simulink model "BatteryFarmTemplate"  (R2022b)
settings: Solver=VariableStepAuto  StartTime=0.0  StopTime=10.0  RelTol=1e-3  AbsTol=1e-3  EnableMultiTasking=on
libraries: ee_lib x242, sdl_lib x84, fl_lib x43
(part 2 of 5)

== system BatteryFarmTemplate/Battery Conex 1/Battery Charger 3 ==
  DC Voltage Source : fl_lib/Electrical/Electrical Sources/DC Voltage Source  v0=24 V
  DC Voltage Source1 : fl_lib/Electrical/Electrical Sources/DC Voltage Source  v0=24 V
  DC Voltage Source2 : fl_lib/Electrical/Electrical Sources/DC Voltage Source  v0=24 V
  SPST Relay : ee_lib/Switches & Breakers/Relays/SPST Relay  block_choices=ee.enum.controlport.ps  R_closed=0.01 Ohm  G_open=1e-8 1/Ohm  Threshold=0  exposemeasurement=ee.enum.exposemeasurement.hidden  V_rated=5 V  V_energize=75  V_deenergize=25  l_winding=0.08 H  r_winding=12.5 Ohm  g_winding=1e-9 1/Ohm  T_brk_C_S=0 s  T_mak_C_S=0 s  enable_faults=ee.enum.relays.enable.no  fault_action=ee.enum.relays.faultaction.none  fault_types=ee.enum.relays.faultTypes.winding  fault_condition_ps=ee.enum.relays.faultConditionSPSTps.csstuck  r_deg_closed_s=1e-9 Ohm  winding_tau_fault=1e-3 s  tau_fault=1e-3 s  enable_temporal_fault=ee.enum.relays.enable.no  t_fault_stick=1 s  t_fault_ComOpen=1 s  t_fault=1 s  enable_behavioral_fault=ee.enum.relays.enable.no  winding_max_permissible_voltage=inf V  n_fail_on_voltage=1  winding_max_permissible_current=inf A  max_permissible_current=inf A  t_fail_on_current=1 s
      settings: InternalSimscapePortConfiguration="{\"Bottom\":[],\"Left\":[{\"id\":\"PS\",\"label\":\"PS\",\"type\":\"input\"}],\"Right\":[{\"id\":\"S\",\"label\":\"S\",\"type\":\"foundation.electrical.electrical\"},{\"id\":\"COM\",\"label\":\"C\",\"type\":\"foundation.electrical.electrical\"}],\"Top\":[]}"
  SPST Relay1 : ee_lib/Switches & Breakers/Relays/SPST Relay  block_choices=ee.enum.controlport.ps  R_closed=0.01 Ohm  G_open=1e-8 1/Ohm  Threshold=0  exposemeasurement=ee.enum.exposemeasurement.hidden  V_rated=5 V  V_energize=75  V_deenergize=25  l_winding=0.08 H  r_winding=12.5 Ohm  g_winding=1e-9 1/Ohm  T_brk_C_S=0 s  T_mak_C_S=0 s  enable_faults=ee.enum.relays.enable.no  fault_action=ee.enum.relays.faultaction.none  fault_types=ee.enum.relays.faultTypes.winding  fault_condition_ps=ee.enum.relays.faultConditionSPSTps.csstuck  r_deg_closed_s=1e-9 Ohm  winding_tau_fault=1e-3 s  tau_fault=1e-3 s  enable_temporal_fault=ee.enum.relays.enable.no  t_fault_stick=1 s  t_fault_ComOpen=1 s  t_fault=1 s  enable_behavioral_fault=ee.enum.relays.enable.no  winding_max_permissible_voltage=inf V  n_fail_on_voltage=1  winding_max_permissible_current=inf A  max_permissible_current=inf A  t_fail_on_current=1 s
      settings: InternalSimscapePortConfiguration="{\"Bottom\":[],\"Left\":[{\"id\":\"PS\",\"label\":\"PS\",\"type\":\"input\"}],\"Right\":[{\"id\":\"S\",\"label\":\"S\",\"type\":\"foundation.electrical.electrical\"},{\"id\":\"COM\",\"label\":\"C\",\"type\":\"foundation.electrical.electrical\"}],\"Top\":[]}"
  SPST Relay2 : ee_lib/Switches & Breakers/Relays/SPST Relay  block_choices=ee.enum.controlport.ps  R_closed=0.01 Ohm  G_open=1e-8 1/Ohm  Threshold=0  exposemeasurement=ee.enum.exposemeasurement.hidden  V_rated=5 V  V_energize=75  V_deenergize=25  l_winding=0.08 H  r_winding=12.5 Ohm  g_winding=1e-9 1/Ohm  T_brk_C_S=0 s  T_mak_C_S=0 s  enable_faults=ee.enum.relays.enable.no  fault_action=ee.enum.relays.faultaction.none  fault_types=ee.enum.relays.faultTypes.winding  fault_condition_ps=ee.enum.relays.faultConditionSPSTps.csstuck  r_deg_closed_s=1e-9 Ohm  winding_tau_fault=1e-3 s  tau_fault=1e-3 s  enable_temporal_fault=ee.enum.relays.enable.no  t_fault_stick=1 s  t_fault_ComOpen=1 s  t_fault=1 s  enable_behavioral_fault=ee.enum.relays.enable.no  winding_max_permissible_voltage=inf V  n_fail_on_voltage=1  winding_max_permissible_current=inf A  max_permissible_current=inf A  t_fail_on_current=1 s
      settings: InternalSimscapePortConfiguration="{\"Bottom\":[],\"Left\":[{\"id\":\"PS\",\"label\":\"PS\",\"type\":\"input\"}],\"Right\":[{\"id\":\"S\",\"label\":\"S\",\"type\":\"foundation.electrical.electrical\"},{\"id\":\"COM\",\"label\":\"C\",\"type\":\"foundation.electrical.electrical\"}],\"Top\":[]}"
  In 1 : PMIOPort  Side=Left
  Out 1 : PMIOPort  Port=2  Side=Left
  In 2 : PMIOPort  Port=3  Side=Left
  Out 2 : PMIOPort  Port=4  Side=Left
  In 3 : PMIOPort  Port=5  Side=Left
  Out 3 : PMIOPort  Port=6  Side=Left
  Energerize Battery Charger : PMIOPort  Port=7  Side=Right
  connections:
  DC Voltage Source/LConn1 -- SPST Relay/RConn1
  SPST Relay/RConn2 -- In 1/RConn1
  DC Voltage Source/RConn1 -- Out 1/RConn1
  DC Voltage Source1/RConn1 -- Out 2/RConn1
  DC Voltage Source1/LConn1 -- SPST Relay1/RConn1
  SPST Relay1/RConn2 -- In 2/RConn1
  DC Voltage Source2/RConn1 -- Out 3/RConn1
  DC Voltage Source2/LConn1 -- SPST Relay2/RConn1
  SPST Relay2/RConn2 -- In 3/RConn1
  SPST Relay1/LConn1 -- Energerize Battery Charger/RConn1 -- SPST Relay/LConn1 -- SPST Relay2/LConn1

== system BatteryFarmTemplate/Battery Conex 1/Battery Charger 4 ==
  DC Voltage Source : fl_lib/Electrical/Electrical Sources/DC Voltage Source  v0=24 V
  DC Voltage Source1 : fl_lib/Electrical/Electrical Sources/DC Voltage Source  v0=24 V
  DC Voltage Source2 : fl_lib/Electrical/Electrical Sources/DC Voltage Source  v0=24 V
  SPST Relay : ee_lib/Switches & Breakers/Relays/SPST Relay  block_choices=ee.enum.controlport.ps  R_closed=0.01 Ohm  G_open=1e-8 1/Ohm  Threshold=0  exposemeasurement=ee.enum.exposemeasurement.hidden  V_rated=5 V  V_energize=75  V_deenergize=25  l_winding=0.08 H  r_winding=12.5 Ohm  g_winding=1e-9 1/Ohm  T_brk_C_S=0 s  T_mak_C_S=0 s  enable_faults=ee.enum.relays.enable.no  fault_action=ee.enum.relays.faultaction.none  fault_types=ee.enum.relays.faultTypes.winding  fault_condition_ps=ee.enum.relays.faultConditionSPSTps.csstuck  r_deg_closed_s=1e-9 Ohm  winding_tau_fault=1e-3 s  tau_fault=1e-3 s  enable_temporal_fault=ee.enum.relays.enable.no  t_fault_stick=1 s  t_fault_ComOpen=1 s  t_fault=1 s  enable_behavioral_fault=ee.enum.relays.enable.no  winding_max_permissible_voltage=inf V  n_fail_on_voltage=1  winding_max_permissible_current=inf A  max_permissible_current=inf A  t_fail_on_current=1 s
      settings: InternalSimscapePortConfiguration="{\"Bottom\":[],\"Left\":[{\"id\":\"PS\",\"label\":\"PS\",\"type\":\"input\"}],\"Right\":[{\"id\":\"S\",\"label\":\"S\",\"type\":\"foundation.electrical.electrical\"},{\"id\":\"COM\",\"label\":\"C\",\"type\":\"foundation.electrical.electrical\"}],\"Top\":[]}"
  SPST Relay1 : ee_lib/Switches & Breakers/Relays/SPST Relay  block_choices=ee.enum.controlport.ps  R_closed=0.01 Ohm  G_open=1e-8 1/Ohm  Threshold=0  exposemeasurement=ee.enum.exposemeasurement.hidden  V_rated=5 V  V_energize=75  V_deenergize=25  l_winding=0.08 H  r_winding=12.5 Ohm  g_winding=1e-9 1/Ohm  T_brk_C_S=0 s  T_mak_C_S=0 s  enable_faults=ee.enum.relays.enable.no  fault_action=ee.enum.relays.faultaction.none  fault_types=ee.enum.relays.faultTypes.winding  fault_condition_ps=ee.enum.relays.faultConditionSPSTps.csstuck  r_deg_closed_s=1e-9 Ohm  winding_tau_fault=1e-3 s  tau_fault=1e-3 s  enable_temporal_fault=ee.enum.relays.enable.no  t_fault_stick=1 s  t_fault_ComOpen=1 s  t_fault=1 s  enable_behavioral_fault=ee.enum.relays.enable.no  winding_max_permissible_voltage=inf V  n_fail_on_voltage=1  winding_max_permissible_current=inf A  max_permissible_current=inf A  t_fail_on_current=1 s
      settings: InternalSimscapePortConfiguration="{\"Bottom\":[],\"Left\":[{\"id\":\"PS\",\"label\":\"PS\",\"type\":\"input\"}],\"Right\":[{\"id\":\"S\",\"label\":\"S\",\"type\":\"foundation.electrical.electrical\"},{\"id\":\"COM\",\"label\":\"C\",\"type\":\"foundation.electrical.electrical\"}],\"Top\":[]}"
  SPST Relay2 : ee_lib/Switches & Breakers/Relays/SPST Relay  block_choices=ee.enum.controlport.ps  R_closed=0.01 Ohm  G_open=1e-8 1/Ohm  Threshold=0  exposemeasurement=ee.enum.exposemeasurement.hidden  V_rated=5 V  V_energize=75  V_deenergize=25  l_winding=0.08 H  r_winding=12.5 Ohm  g_winding=1e-9 1/Ohm  T_brk_C_S=0 s  T_mak_C_S=0 s  enable_faults=ee.enum.relays.enable.no  fault_action=ee.enum.relays.faultaction.none  fault_types=ee.enum.relays.faultTypes.winding  fault_condition_ps=ee.enum.relays.faultConditionSPSTps.csstuck  r_deg_closed_s=1e-9 Ohm  winding_tau_fault=1e-3 s  tau_fault=1e-3 s  enable_temporal_fault=ee.enum.relays.enable.no  t_fault_stick=1 s  t_fault_ComOpen=1 s  t_fault=1 s  enable_behavioral_fault=ee.enum.relays.enable.no  winding_max_permissible_voltage=inf V  n_fail_on_voltage=1  winding_max_permissible_current=inf A  max_permissible_current=inf A  t_fail_on_current=1 s
      settings: InternalSimscapePortConfiguration="{\"Bottom\":[],\"Left\":[{\"id\":\"PS\",\"label\":\"PS\",\"type\":\"input\"}],\"Right\":[{\"id\":\"S\",\"label\":\"S\",\"type\":\"foundation.electrical.electrical\"},{\"id\":\"COM\",\"label\":\"C\",\"type\":\"foundation.electrical.electrical\"}],\"Top\":[]}"
  In 1 : PMIOPort  Side=Left
  Out 1 : PMIOPort  Port=2  Side=Left
  In 2 : PMIOPort  Port=3  Side=Left
  Out 2 : PMIOPort  Port=4  Side=Left
  In 3 : PMIOPort  Port=5  Side=Left
  Out 3 : PMIOPort  Port=6  Side=Left
  Energerize Battery Charger : PMIOPort  Port=7  Side=Right
  connections:
  DC Voltage Source/LConn1 -- SPST Relay/RConn1
  SPST Relay/RConn2 -- In 1/RConn1
  DC Voltage Source/RConn1 -- Out 1/RConn1
  DC Voltage Source1/RConn1 -- Out 2/RConn1
  DC Voltage Source1/LConn1 -- SPST Relay1/RConn1
  SPST Relay1/RConn2 -- In 2/RConn1
  DC Voltage Source2/RConn1 -- Out 3/RConn1
  DC Voltage Source2/LConn1 -- SPST Relay2/RConn1
  SPST Relay2/RConn2 -- In 3/RConn1
  SPST Relay1/LConn1 -- Energerize Battery Charger/RConn1 -- SPST Relay/LConn1 -- SPST Relay2/LConn1

== system BatteryFarmTemplate/Battery Conex 1/Battery Charger 5 ==
  DC Voltage Source : fl_lib/Electrical/Electrical Sources/DC Voltage Source  v0=24 V
  DC Voltage Source1 : fl_lib/Electrical/Electrical Sources/DC Voltage Source  v0=24 V
  DC Voltage Source2 : fl_lib/Electrical/Electrical Sources/DC Voltage Source  v0=24 V
  SPST Relay : ee_lib/Switches & Breakers/Relays/SPST Relay  block_choices=ee.enum.controlport.ps  R_closed=0.01 Ohm  G_open=1e-8 1/Ohm  Threshold=0  exposemeasurement=ee.enum.exposemeasurement.hidden  V_rated=5 V  V_energize=75  V_deenergize=25  l_winding=0.08 H  r_winding=12.5 Ohm  g_winding=1e-9 1/Ohm  T_brk_C_S=0 s  T_mak_C_S=0 s  enable_faults=ee.enum.relays.enable.no  fault_action=ee.enum.relays.faultaction.none  fault_types=ee.enum.relays.faultTypes.winding  fault_condition_ps=ee.enum.relays.faultConditionSPSTps.csstuck  r_deg_closed_s=1e-9 Ohm  winding_tau_fault=1e-3 s  tau_fault=1e-3 s  enable_temporal_fault=ee.enum.relays.enable.no  t_fault_stick=1 s  t_fault_ComOpen=1 s  t_fault=1 s  enable_behavioral_fault=ee.enum.relays.enable.no  winding_max_permissible_voltage=inf V  n_fail_on_voltage=1  winding_max_permissible_current=inf A  max_permissible_current=inf A  t_fail_on_current=1 s
      settings: InternalSimscapePortConfiguration="{\"Bottom\":[],\"Left\":[{\"id\":\"PS\",\"label\":\"PS\",\"type\":\"input\"}],\"Right\":[{\"id\":\"S\",\"label\":\"S\",\"type\":\"foundation.electrical.electrical\"},{\"id\":\"COM\",\"label\":\"C\",\"type\":\"foundation.electrical.electrical\"}],\"Top\":[]}"
  SPST Relay1 : ee_lib/Switches & Breakers/Relays/SPST Relay  block_choices=ee.enum.controlport.ps  R_closed=0.01 Ohm  G_open=1e-8 1/Ohm  Threshold=0  exposemeasurement=ee.enum.exposemeasurement.hidden  V_rated=5 V  V_energize=75  V_deenergize=25  l_winding=0.08 H  r_winding=12.5 Ohm  g_winding=1e-9 1/Ohm  T_brk_C_S=0 s  T_mak_C_S=0 s  enable_faults=ee.enum.relays.enable.no  fault_action=ee.enum.relays.faultaction.none  fault_types=ee.enum.relays.faultTypes.winding  fault_condition_ps=ee.enum.relays.faultConditionSPSTps.csstuck  r_deg_closed_s=1e-9 Ohm  winding_tau_fault=1e-3 s  tau_fault=1e-3 s  enable_temporal_fault=ee.enum.relays.enable.no  t_fault_stick=1 s  t_fault_ComOpen=1 s  t_fault=1 s  enable_behavioral_fault=ee.enum.relays.enable.no  winding_max_permissible_voltage=inf V  n_fail_on_voltage=1  winding_max_permissible_current=inf A  max_permissible_current=inf A  t_fail_on_current=1 s
      settings: InternalSimscapePortConfiguration="{\"Bottom\":[],\"Left\":[{\"id\":\"PS\",\"label\":\"PS\",\"type\":\"input\"}],\"Right\":[{\"id\":\"S\",\"label\":\"S\",\"type\":\"foundation.electrical.electrical\"},{\"id\":\"COM\",\"label\":\"C\",\"type\":\"foundation.electrical.electrical\"}],\"Top\":[]}"
  SPST Relay2 : ee_lib/Switches & Breakers/Relays/SPST Relay  block_choices=ee.enum.controlport.ps  R_closed=0.01 Ohm  G_open=1e-8 1/Ohm  Threshold=0  exposemeasurement=ee.enum.exposemeasurement.hidden  V_rated=5 V  V_energize=75  V_deenergize=25  l_winding=0.08 H  r_winding=12.5 Ohm  g_winding=1e-9 1/Ohm  T_brk_C_S=0 s  T_mak_C_S=0 s  enable_faults=ee.enum.relays.enable.no  fault_action=ee.enum.relays.faultaction.none  fault_types=ee.enum.relays.faultTypes.winding  fault_condition_ps=ee.enum.relays.faultConditionSPSTps.csstuck  r_deg_closed_s=1e-9 Ohm  winding_tau_fault=1e-3 s  tau_fault=1e-3 s  enable_temporal_fault=ee.enum.relays.enable.no  t_fault_stick=1 s  t_fault_ComOpen=1 s  t_fault=1 s  enable_behavioral_fault=ee.enum.relays.enable.no  winding_max_permissible_voltage=inf V  n_fail_on_voltage=1  winding_max_permissible_current=inf A  max_permissible_current=inf A  t_fail_on_current=1 s
      settings: InternalSimscapePortConfiguration="{\"Bottom\":[],\"Left\":[{\"id\":\"PS\",\"label\":\"PS\",\"type\":\"input\"}],\"Right\":[{\"id\":\"S\",\"label\":\"S\",\"type\":\"foundation.electrical.electrical\"},{\"id\":\"COM\",\"label\":\"C\",\"type\":\"foundation.electrical.electrical\"}],\"Top\":[]}"
  In 1 : PMIOPort  Side=Left
  Out 1 : PMIOPort  Port=2  Side=Left
  In 2 : PMIOPort  Port=3  Side=Left
  Out 2 : PMIOPort  Port=4  Side=Left
  In 3 : PMIOPort  Port=5  Side=Left
  Out 3 : PMIOPort  Port=6  Side=Left
  Energerize Battery Charger : PMIOPort  Port=7  Side=Right
  connections:
  DC Voltage Source/LConn1 -- SPST Relay/RConn1
  SPST Relay/RConn2 -- In 1/RConn1
  DC Voltage Source/RConn1 -- Out 1/RConn1
  DC Voltage Source1/RConn1 -- Out 2/RConn1
  DC Voltage Source1/LConn1 -- SPST Relay1/RConn1
  SPST Relay1/RConn2 -- In 2/RConn1
  DC Voltage Source2/RConn1 -- Out 3/RConn1
  DC Voltage Source2/LConn1 -- SPST Relay2/RConn1
  SPST Relay2/RConn2 -- In 3/RConn1
  SPST Relay1/LConn1 -- Energerize Battery Charger/RConn1 -- SPST Relay/LConn1 -- SPST Relay2/LConn1

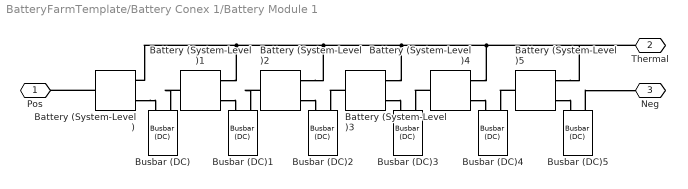
== system BatteryFarmTemplate/Battery Conex 1/Battery Module 1 ==
  Battery (System-Level){,1..5} (6 alike) : sdl_lib/Sources/Battery (System-Level)  Vnom=3.1 V  R1=0.021 Ohm  prm_AH=sdl.enum.InfiniteFinite.Infinite  AH=50 A*hr  V1=11.5 V  AH1=25 A*hr  prm_R2=sdl.enum.DisabledEnabled.Disabled  R2=2000 Ohm  thermal_port=simscape.enum.thermaleffects.model  thermal_mass=30000 J/K  i_specify=off  i_priority=None  i=0 A  i_nominal_specify=off  i_nominal_unit=A  i_nominal_value=1  v_specify=off  v_priority=None  v=0 V  v_nominal_specify=off  v_nominal_unit=V  v_nominal_value=1  charge_specify=off  charge_priority=High  charge=50 A*hr  charge_nominal_specify=off  charge_nominal_unit=A*hr  charge_nominal_value=1  temperature_specify=off  temperature_priority=High  temperature=300 K  temperature_nominal_specify=off  temperature_nominal_unit=K  temperature_nominal_value=1
      settings: InternalSimscapePortConfiguration="{\"Bottom\":[],\"Left\":[{\"id\":\"p\",\"label\":\"+\",\"type\":\"foundation.electrical.electrical\"}],\"Right\":[{\"id\":\"n\",\"label\":\"-\",\"type\":\"foundation.electrical.electrical\"},{\"id\":\"H\",\"label\":\"H\",\"type\":\"foundation.thermal.thermal\"}],\"Top\":[]}"
  Busbar (DC){,1..5} (6 alike) : ee_lib/Connectors & References/Busbar (DC)  n_nodes=ee.enum.connectors.busbar_number_of_connections.one  VRated=1e3 V  measurement_type=ee.enum.measurementType.instantaneous  averaging_period=1e-2 s  show_ps=ee.enum.connectors.busbar_measurement.false
      settings: InternalSimscapePortConfiguration="{\"Bottom\":[],\"Left\":[{\"id\":\"p1\",\"label\":\"1+\",\"type\":\"foundation.electrical.electrical\"},{\"id\":\"n1\",\"label\":\"1-\",\"type\":\"foundation.electrical.electrical\"}],\"Right\":[],\"Top\":[]}"
  Pos : PMIOPort  Side=Left
  Thermal : PMIOPort  Port=2  Side=Right
  Neg : PMIOPort  Port=3  Side=Right
  connections:
  Battery (System-Level)3/RConn1 -- Busbar (DC)3/LConn1
  Battery (System-Level)1/RConn1 -- Busbar (DC)1/LConn1
  Battery (System-Level)1/RConn2 -- Battery (System-Level)2/RConn2 -- Battery (System-Level)3/RConn2 -- Battery (System-Level)4/RConn2 -- Battery (System-Level)5/RConn2 -- Thermal/RConn1 -- Battery (System-Level)/RConn2
  Battery (System-Level)3/LConn1 -- Busbar (DC)2/LConn2
  Battery (System-Level)5/RConn1 -- Busbar (DC)5/LConn1
  Battery (System-Level)/RConn1 -- Busbar (DC)/LConn1
  Battery (System-Level)4/LConn1 -- Busbar (DC)3/LConn2
  Battery (System-Level)2/RConn1 -- Busbar (DC)2/LConn1
  Busbar (DC)5/LConn2 -- Neg/RConn1
  Battery (System-Level)/LConn1 -- Pos/RConn1
  Battery (System-Level)2/LConn1 -- Busbar (DC)1/LConn2
  Battery (System-Level)4/RConn1 -- Busbar (DC)4/LConn1
  Battery (System-Level)5/LConn1 -- Busbar (DC)4/LConn2
  Battery (System-Level)1/LConn1 -- Busbar (DC)/LConn2

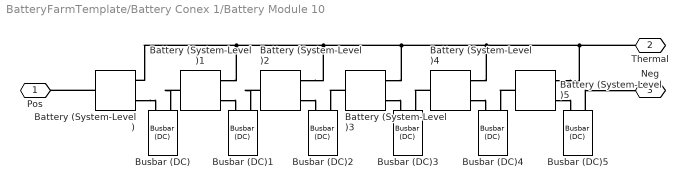
== system BatteryFarmTemplate/Battery Conex 1/Battery Module 10 ==
  Battery (System-Level){,1..5} (6 alike) : sdl_lib/Sources/Battery (System-Level)  Vnom=3.1 V  R1=0.021 Ohm  prm_AH=sdl.enum.InfiniteFinite.Infinite  AH=50 A*hr  V1=11.5 V  AH1=25 A*hr  prm_R2=sdl.enum.DisabledEnabled.Disabled  R2=2000 Ohm  thermal_port=simscape.enum.thermaleffects.model  thermal_mass=30000 J/K  i_specify=off  i_priority=None  i=0 A  i_nominal_specify=off  i_nominal_unit=A  i_nominal_value=1  v_specify=off  v_priority=None  v=0 V  v_nominal_specify=off  v_nominal_unit=V  v_nominal_value=1  charge_specify=off  charge_priority=High  charge=50 A*hr  charge_nominal_specify=off  charge_nominal_unit=A*hr  charge_nominal_value=1  temperature_specify=off  temperature_priority=High  temperature=300 K  temperature_nominal_specify=off  temperature_nominal_unit=K  temperature_nominal_value=1
      settings: InternalSimscapePortConfiguration="{\"Bottom\":[],\"Left\":[{\"id\":\"p\",\"label\":\"+\",\"type\":\"foundation.electrical.electrical\"}],\"Right\":[{\"id\":\"n\",\"label\":\"-\",\"type\":\"foundation.electrical.electrical\"},{\"id\":\"H\",\"label\":\"H\",\"type\":\"foundation.thermal.thermal\"}],\"Top\":[]}"
  Busbar (DC){,1..5} (6 alike) : ee_lib/Connectors & References/Busbar (DC)  n_nodes=ee.enum.connectors.busbar_number_of_connections.one  VRated=1e3 V  measurement_type=ee.enum.measurementType.instantaneous  averaging_period=1e-2 s  show_ps=ee.enum.connectors.busbar_measurement.false
      settings: InternalSimscapePortConfiguration="{\"Bottom\":[],\"Left\":[{\"id\":\"p1\",\"label\":\"1+\",\"type\":\"foundation.electrical.electrical\"},{\"id\":\"n1\",\"label\":\"1-\",\"type\":\"foundation.electrical.electrical\"}],\"Right\":[],\"Top\":[]}"
  Pos : PMIOPort  Side=Left
  Thermal : PMIOPort  Port=2  Side=Right
  Neg : PMIOPort  Port=3  Side=Right
  connections:
  Battery (System-Level)3/RConn1 -- Busbar (DC)3/LConn1
  Battery (System-Level)1/RConn1 -- Busbar (DC)1/LConn1
  Battery (System-Level)5/RConn2 -- Battery (System-Level)4/RConn2 -- Battery (System-Level)3/RConn2 -- Battery (System-Level)2/RConn2 -- Battery (System-Level)1/RConn2 -- Battery (System-Level)/RConn2 -- Thermal/RConn1
  Battery (System-Level)3/LConn1 -- Busbar (DC)2/LConn2
  Battery (System-Level)5/RConn1 -- Busbar (DC)5/LConn1
  Battery (System-Level)/RConn1 -- Busbar (DC)/LConn1
  Battery (System-Level)4/LConn1 -- Busbar (DC)3/LConn2
  Battery (System-Level)2/RConn1 -- Busbar (DC)2/LConn1
  Busbar (DC)5/LConn2 -- Neg/RConn1
  Battery (System-Level)/LConn1 -- Pos/RConn1
  Battery (System-Level)2/LConn1 -- Busbar (DC)1/LConn2
  Battery (System-Level)4/RConn1 -- Busbar (DC)4/LConn1
  Battery (System-Level)5/LConn1 -- Busbar (DC)4/LConn2
  Battery (System-Level)1/LConn1 -- Busbar (DC)/LConn2

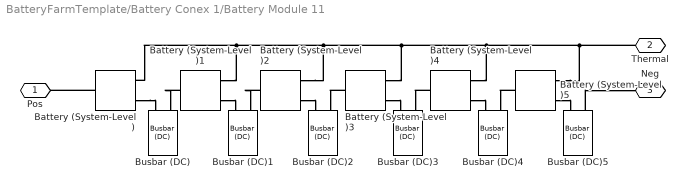
== system BatteryFarmTemplate/Battery Conex 1/Battery Module 11 ==
  Battery (System-Level){,1..5} (6 alike) : sdl_lib/Sources/Battery (System-Level)  Vnom=3.1 V  R1=0.021 Ohm  prm_AH=sdl.enum.InfiniteFinite.Infinite  AH=50 A*hr  V1=11.5 V  AH1=25 A*hr  prm_R2=sdl.enum.DisabledEnabled.Disabled  R2=2000 Ohm  thermal_port=simscape.enum.thermaleffects.model  thermal_mass=30000 J/K  i_specify=off  i_priority=None  i=0 A  i_nominal_specify=off  i_nominal_unit=A  i_nominal_value=1  v_specify=off  v_priority=None  v=0 V  v_nominal_specify=off  v_nominal_unit=V  v_nominal_value=1  charge_specify=off  charge_priority=High  charge=50 A*hr  charge_nominal_specify=off  charge_nominal_unit=A*hr  charge_nominal_value=1  temperature_specify=off  temperature_priority=High  temperature=300 K  temperature_nominal_specify=off  temperature_nominal_unit=K  temperature_nominal_value=1
      settings: InternalSimscapePortConfiguration="{\"Bottom\":[],\"Left\":[{\"id\":\"p\",\"label\":\"+\",\"type\":\"foundation.electrical.electrical\"}],\"Right\":[{\"id\":\"n\",\"label\":\"-\",\"type\":\"foundation.electrical.electrical\"},{\"id\":\"H\",\"label\":\"H\",\"type\":\"foundation.thermal.thermal\"}],\"Top\":[]}"
  Busbar (DC){,1..5} (6 alike) : ee_lib/Connectors & References/Busbar (DC)  n_nodes=ee.enum.connectors.busbar_number_of_connections.one  VRated=1e3 V  measurement_type=ee.enum.measurementType.instantaneous  averaging_period=1e-2 s  show_ps=ee.enum.connectors.busbar_measurement.false
      settings: InternalSimscapePortConfiguration="{\"Bottom\":[],\"Left\":[{\"id\":\"p1\",\"label\":\"1+\",\"type\":\"foundation.electrical.electrical\"},{\"id\":\"n1\",\"label\":\"1-\",\"type\":\"foundation.electrical.electrical\"}],\"Right\":[],\"Top\":[]}"
  Pos : PMIOPort  Side=Left
  Thermal : PMIOPort  Port=2  Side=Right
  Neg : PMIOPort  Port=3  Side=Right
  connections:
  Battery (System-Level)3/RConn1 -- Busbar (DC)3/LConn1
  Battery (System-Level)1/RConn1 -- Busbar (DC)1/LConn1
  Battery (System-Level)5/RConn2 -- Battery (System-Level)4/RConn2 -- Battery (System-Level)3/RConn2 -- Battery (System-Level)2/RConn2 -- Battery (System-Level)1/RConn2 -- Battery (System-Level)/RConn2 -- Thermal/RConn1
  Battery (System-Level)3/LConn1 -- Busbar (DC)2/LConn2
  Battery (System-Level)5/RConn1 -- Busbar (DC)5/LConn1
  Battery (System-Level)/RConn1 -- Busbar (DC)/LConn1
  Battery (System-Level)4/LConn1 -- Busbar (DC)3/LConn2
  Battery (System-Level)2/RConn1 -- Busbar (DC)2/LConn1
  Busbar (DC)5/LConn2 -- Neg/RConn1
  Battery (System-Level)/LConn1 -- Pos/RConn1
  Battery (System-Level)2/LConn1 -- Busbar (DC)1/LConn2
  Battery (System-Level)4/RConn1 -- Busbar (DC)4/LConn1
  Battery (System-Level)5/LConn1 -- Busbar (DC)4/LConn2
  Battery (System-Level)1/LConn1 -- Busbar (DC)/LConn2

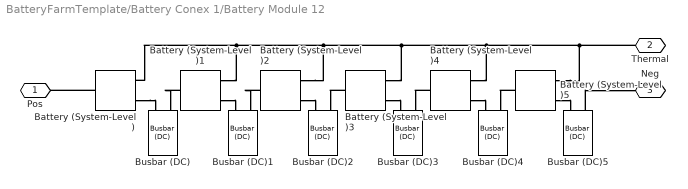
== system BatteryFarmTemplate/Battery Conex 1/Battery Module 12 ==
  Battery (System-Level){,1..5} (6 alike) : sdl_lib/Sources/Battery (System-Level)  Vnom=3.1 V  R1=0.021 Ohm  prm_AH=sdl.enum.InfiniteFinite.Infinite  AH=50 A*hr  V1=11.5 V  AH1=25 A*hr  prm_R2=sdl.enum.DisabledEnabled.Disabled  R2=2000 Ohm  thermal_port=simscape.enum.thermaleffects.model  thermal_mass=30000 J/K  i_specify=off  i_priority=None  i=0 A  i_nominal_specify=off  i_nominal_unit=A  i_nominal_value=1  v_specify=off  v_priority=None  v=0 V  v_nominal_specify=off  v_nominal_unit=V  v_nominal_value=1  charge_specify=off  charge_priority=High  charge=50 A*hr  charge_nominal_specify=off  charge_nominal_unit=A*hr  charge_nominal_value=1  temperature_specify=off  temperature_priority=High  temperature=300 K  temperature_nominal_specify=off  temperature_nominal_unit=K  temperature_nominal_value=1
      settings: InternalSimscapePortConfiguration="{\"Bottom\":[],\"Left\":[{\"id\":\"p\",\"label\":\"+\",\"type\":\"foundation.electrical.electrical\"}],\"Right\":[{\"id\":\"n\",\"label\":\"-\",\"type\":\"foundation.electrical.electrical\"},{\"id\":\"H\",\"label\":\"H\",\"type\":\"foundation.thermal.thermal\"}],\"Top\":[]}"
  Busbar (DC){,1..5} (6 alike) : ee_lib/Connectors & References/Busbar (DC)  n_nodes=ee.enum.connectors.busbar_number_of_connections.one  VRated=1e3 V  measurement_type=ee.enum.measurementType.instantaneous  averaging_period=1e-2 s  show_ps=ee.enum.connectors.busbar_measurement.false
      settings: InternalSimscapePortConfiguration="{\"Bottom\":[],\"Left\":[{\"id\":\"p1\",\"label\":\"1+\",\"type\":\"foundation.electrical.electrical\"},{\"id\":\"n1\",\"label\":\"1-\",\"type\":\"foundation.electrical.electrical\"}],\"Right\":[],\"Top\":[]}"
  Pos : PMIOPort  Side=Left
  Thermal : PMIOPort  Port=2  Side=Right
  Neg : PMIOPort  Port=3  Side=Right
  connections:
  Battery (System-Level)3/RConn1 -- Busbar (DC)3/LConn1
  Battery (System-Level)1/RConn1 -- Busbar (DC)1/LConn1
  Battery (System-Level)5/RConn2 -- Battery (System-Level)4/RConn2 -- Battery (System-Level)3/RConn2 -- Battery (System-Level)2/RConn2 -- Battery (System-Level)1/RConn2 -- Battery (System-Level)/RConn2 -- Thermal/RConn1
  Battery (System-Level)3/LConn1 -- Busbar (DC)2/LConn2
  Battery (System-Level)5/RConn1 -- Busbar (DC)5/LConn1
  Battery (System-Level)/RConn1 -- Busbar (DC)/LConn1
  Battery (System-Level)4/LConn1 -- Busbar (DC)3/LConn2
  Battery (System-Level)2/RConn1 -- Busbar (DC)2/LConn1
  Busbar (DC)5/LConn2 -- Neg/RConn1
  Battery (System-Level)/LConn1 -- Pos/RConn1
  Battery (System-Level)2/LConn1 -- Busbar (DC)1/LConn2
  Battery (System-Level)4/RConn1 -- Busbar (DC)4/LConn1
  Battery (System-Level)5/LConn1 -- Busbar (DC)4/LConn2
  Battery (System-Level)1/LConn1 -- Busbar (DC)/LConn2

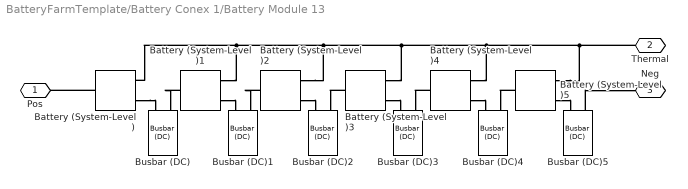
== system BatteryFarmTemplate/Battery Conex 1/Battery Module 13 ==
  Battery (System-Level){,1..5} (6 alike) : sdl_lib/Sources/Battery (System-Level)  Vnom=3.1 V  R1=0.021 Ohm  prm_AH=sdl.enum.InfiniteFinite.Infinite  AH=50 A*hr  V1=11.5 V  AH1=25 A*hr  prm_R2=sdl.enum.DisabledEnabled.Disabled  R2=2000 Ohm  thermal_port=simscape.enum.thermaleffects.model  thermal_mass=30000 J/K  i_specify=off  i_priority=None  i=0 A  i_nominal_specify=off  i_nominal_unit=A  i_nominal_value=1  v_specify=off  v_priority=None  v=0 V  v_nominal_specify=off  v_nominal_unit=V  v_nominal_value=1  charge_specify=off  charge_priority=High  charge=50 A*hr  charge_nominal_specify=off  charge_nominal_unit=A*hr  charge_nominal_value=1  temperature_specify=off  temperature_priority=High  temperature=300 K  temperature_nominal_specify=off  temperature_nominal_unit=K  temperature_nominal_value=1
      settings: InternalSimscapePortConfiguration="{\"Bottom\":[],\"Left\":[{\"id\":\"p\",\"label\":\"+\",\"type\":\"foundation.electrical.electrical\"}],\"Right\":[{\"id\":\"n\",\"label\":\"-\",\"type\":\"foundation.electrical.electrical\"},{\"id\":\"H\",\"label\":\"H\",\"type\":\"foundation.thermal.thermal\"}],\"Top\":[]}"
  Busbar (DC){,1..5} (6 alike) : ee_lib/Connectors & References/Busbar (DC)  n_nodes=ee.enum.connectors.busbar_number_of_connections.one  VRated=1e3 V  measurement_type=ee.enum.measurementType.instantaneous  averaging_period=1e-2 s  show_ps=ee.enum.connectors.busbar_measurement.false
      settings: InternalSimscapePortConfiguration="{\"Bottom\":[],\"Left\":[{\"id\":\"p1\",\"label\":\"1+\",\"type\":\"foundation.electrical.electrical\"},{\"id\":\"n1\",\"label\":\"1-\",\"type\":\"foundation.electrical.electrical\"}],\"Right\":[],\"Top\":[]}"
  Pos : PMIOPort  Side=Left
  Thermal : PMIOPort  Port=2  Side=Right
  Neg : PMIOPort  Port=3  Side=Right
  connections:
  Battery (System-Level)3/RConn1 -- Busbar (DC)3/LConn1
  Battery (System-Level)1/RConn1 -- Busbar (DC)1/LConn1
  Battery (System-Level)5/RConn2 -- Battery (System-Level)4/RConn2 -- Battery (System-Level)3/RConn2 -- Battery (System-Level)2/RConn2 -- Battery (System-Level)1/RConn2 -- Battery (System-Level)/RConn2 -- Thermal/RConn1
  Battery (System-Level)3/LConn1 -- Busbar (DC)2/LConn2
  Battery (System-Level)5/RConn1 -- Busbar (DC)5/LConn1
  Battery (System-Level)/RConn1 -- Busbar (DC)/LConn1
  Battery (System-Level)4/LConn1 -- Busbar (DC)3/LConn2
  Battery (System-Level)2/RConn1 -- Busbar (DC)2/LConn1
  Busbar (DC)5/LConn2 -- Neg/RConn1
  Battery (System-Level)/LConn1 -- Pos/RConn1
  Battery (System-Level)2/LConn1 -- Busbar (DC)1/LConn2
  Battery (System-Level)4/RConn1 -- Busbar (DC)4/LConn1
  Battery (System-Level)5/LConn1 -- Busbar (DC)4/LConn2
  Battery (System-Level)1/LConn1 -- Busbar (DC)/LConn2

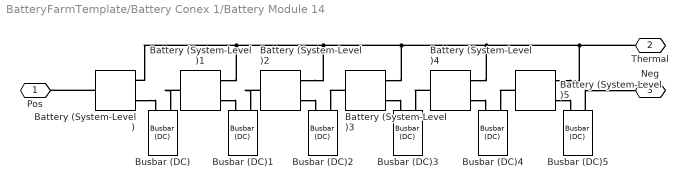
== system BatteryFarmTemplate/Battery Conex 1/Battery Module 14 ==
  Battery (System-Level){,1..5} (6 alike) : sdl_lib/Sources/Battery (System-Level)  Vnom=3.1 V  R1=0.021 Ohm  prm_AH=sdl.enum.InfiniteFinite.Infinite  AH=50 A*hr  V1=11.5 V  AH1=25 A*hr  prm_R2=sdl.enum.DisabledEnabled.Disabled  R2=2000 Ohm  thermal_port=simscape.enum.thermaleffects.model  thermal_mass=30000 J/K  i_specify=off  i_priority=None  i=0 A  i_nominal_specify=off  i_nominal_unit=A  i_nominal_value=1  v_specify=off  v_priority=None  v=0 V  v_nominal_specify=off  v_nominal_unit=V  v_nominal_value=1  charge_specify=off  charge_priority=High  charge=50 A*hr  charge_nominal_specify=off  charge_nominal_unit=A*hr  charge_nominal_value=1  temperature_specify=off  temperature_priority=High  temperature=300 K  temperature_nominal_specify=off  temperature_nominal_unit=K  temperature_nominal_value=1
      settings: InternalSimscapePortConfiguration="{\"Bottom\":[],\"Left\":[{\"id\":\"p\",\"label\":\"+\",\"type\":\"foundation.electrical.electrical\"}],\"Right\":[{\"id\":\"n\",\"label\":\"-\",\"type\":\"foundation.electrical.electrical\"},{\"id\":\"H\",\"label\":\"H\",\"type\":\"foundation.thermal.thermal\"}],\"Top\":[]}"
  Busbar (DC){,1..5} (6 alike) : ee_lib/Connectors & References/Busbar (DC)  n_nodes=ee.enum.connectors.busbar_number_of_connections.one  VRated=1e3 V  measurement_type=ee.enum.measurementType.instantaneous  averaging_period=1e-2 s  show_ps=ee.enum.connectors.busbar_measurement.false
      settings: InternalSimscapePortConfiguration="{\"Bottom\":[],\"Left\":[{\"id\":\"p1\",\"label\":\"1+\",\"type\":\"foundation.electrical.electrical\"},{\"id\":\"n1\",\"label\":\"1-\",\"type\":\"foundation.electrical.electrical\"}],\"Right\":[],\"Top\":[]}"
  Pos : PMIOPort  Side=Left
  Thermal : PMIOPort  Port=2  Side=Right
  Neg : PMIOPort  Port=3  Side=Right
  connections:
  Battery (System-Level)3/RConn1 -- Busbar (DC)3/LConn1
  Battery (System-Level)1/RConn1 -- Busbar (DC)1/LConn1
  Battery (System-Level)5/RConn2 -- Battery (System-Level)4/RConn2 -- Battery (System-Level)3/RConn2 -- Battery (System-Level)2/RConn2 -- Battery (System-Level)1/RConn2 -- Battery (System-Level)/RConn2 -- Thermal/RConn1
  Battery (System-Level)3/LConn1 -- Busbar (DC)2/LConn2
  Battery (System-Level)5/RConn1 -- Busbar (DC)5/LConn1
  Battery (System-Level)/RConn1 -- Busbar (DC)/LConn1
  Battery (System-Level)4/LConn1 -- Busbar (DC)3/LConn2
  Battery (System-Level)2/RConn1 -- Busbar (DC)2/LConn1
  Busbar (DC)5/LConn2 -- Neg/RConn1
  Battery (System-Level)/LConn1 -- Pos/RConn1
  Battery (System-Level)2/LConn1 -- Busbar (DC)1/LConn2
  Battery (System-Level)4/RConn1 -- Busbar (DC)4/LConn1
  Battery (System-Level)5/LConn1 -- Busbar (DC)4/LConn2
  Battery (System-Level)1/LConn1 -- Busbar (DC)/LConn2

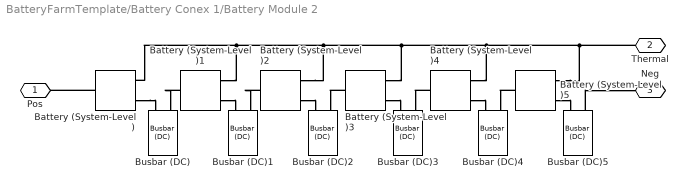
== system BatteryFarmTemplate/Battery Conex 1/Battery Module 2 ==
  Battery (System-Level){,1..5} (6 alike) : sdl_lib/Sources/Battery (System-Level)  Vnom=3.1 V  R1=0.021 Ohm  prm_AH=sdl.enum.InfiniteFinite.Infinite  AH=50 A*hr  V1=11.5 V  AH1=25 A*hr  prm_R2=sdl.enum.DisabledEnabled.Disabled  R2=2000 Ohm  thermal_port=simscape.enum.thermaleffects.model  thermal_mass=30000 J/K  i_specify=off  i_priority=None  i=0 A  i_nominal_specify=off  i_nominal_unit=A  i_nominal_value=1  v_specify=off  v_priority=None  v=0 V  v_nominal_specify=off  v_nominal_unit=V  v_nominal_value=1  charge_specify=off  charge_priority=High  charge=50 A*hr  charge_nominal_specify=off  charge_nominal_unit=A*hr  charge_nominal_value=1  temperature_specify=off  temperature_priority=High  temperature=300 K  temperature_nominal_specify=off  temperature_nominal_unit=K  temperature_nominal_value=1
      settings: InternalSimscapePortConfiguration="{\"Bottom\":[],\"Left\":[{\"id\":\"p\",\"label\":\"+\",\"type\":\"foundation.electrical.electrical\"}],\"Right\":[{\"id\":\"n\",\"label\":\"-\",\"type\":\"foundation.electrical.electrical\"},{\"id\":\"H\",\"label\":\"H\",\"type\":\"foundation.thermal.thermal\"}],\"Top\":[]}"
  Busbar (DC){,1..5} (6 alike) : ee_lib/Connectors & References/Busbar (DC)  n_nodes=ee.enum.connectors.busbar_number_of_connections.one  VRated=1e3 V  measurement_type=ee.enum.measurementType.instantaneous  averaging_period=1e-2 s  show_ps=ee.enum.connectors.busbar_measurement.false
      settings: InternalSimscapePortConfiguration="{\"Bottom\":[],\"Left\":[{\"id\":\"p1\",\"label\":\"1+\",\"type\":\"foundation.electrical.electrical\"},{\"id\":\"n1\",\"label\":\"1-\",\"type\":\"foundation.electrical.electrical\"}],\"Right\":[],\"Top\":[]}"
  Pos : PMIOPort  Side=Left
  Thermal : PMIOPort  Port=2  Side=Right
  Neg : PMIOPort  Port=3  Side=Right
  connections:
  Battery (System-Level)3/RConn1 -- Busbar (DC)3/LConn1
  Battery (System-Level)1/RConn1 -- Busbar (DC)1/LConn1
  Battery (System-Level)5/RConn2 -- Battery (System-Level)4/RConn2 -- Battery (System-Level)3/RConn2 -- Battery (System-Level)2/RConn2 -- Battery (System-Level)1/RConn2 -- Battery (System-Level)/RConn2 -- Thermal/RConn1
  Battery (System-Level)3/LConn1 -- Busbar (DC)2/LConn2
  Battery (System-Level)5/RConn1 -- Busbar (DC)5/LConn1
  Battery (System-Level)/RConn1 -- Busbar (DC)/LConn1
  Battery (System-Level)4/LConn1 -- Busbar (DC)3/LConn2
  Battery (System-Level)2/RConn1 -- Busbar (DC)2/LConn1
  Busbar (DC)5/LConn2 -- Neg/RConn1
  Battery (System-Level)/LConn1 -- Pos/RConn1
  Battery (System-Level)2/LConn1 -- Busbar (DC)1/LConn2
  Battery (System-Level)4/RConn1 -- Busbar (DC)4/LConn1
  Battery (System-Level)5/LConn1 -- Busbar (DC)4/LConn2
  Battery (System-Level)1/LConn1 -- Busbar (DC)/LConn2

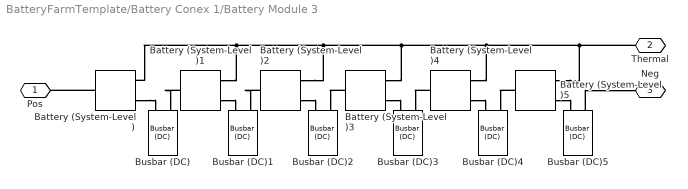
== system BatteryFarmTemplate/Battery Conex 1/Battery Module 3 ==
  Battery (System-Level){,1..5} (6 alike) : sdl_lib/Sources/Battery (System-Level)  Vnom=3.1 V  R1=0.021 Ohm  prm_AH=sdl.enum.InfiniteFinite.Infinite  AH=50 A*hr  V1=11.5 V  AH1=25 A*hr  prm_R2=sdl.enum.DisabledEnabled.Disabled  R2=2000 Ohm  thermal_port=simscape.enum.thermaleffects.model  thermal_mass=30000 J/K  i_specify=off  i_priority=None  i=0 A  i_nominal_specify=off  i_nominal_unit=A  i_nominal_value=1  v_specify=off  v_priority=None  v=0 V  v_nominal_specify=off  v_nominal_unit=V  v_nominal_value=1  charge_specify=off  charge_priority=High  charge=50 A*hr  charge_nominal_specify=off  charge_nominal_unit=A*hr  charge_nominal_value=1  temperature_specify=off  temperature_priority=High  temperature=300 K  temperature_nominal_specify=off  temperature_nominal_unit=K  temperature_nominal_value=1
      settings: InternalSimscapePortConfiguration="{\"Bottom\":[],\"Left\":[{\"id\":\"p\",\"label\":\"+\",\"type\":\"foundation.electrical.electrical\"}],\"Right\":[{\"id\":\"n\",\"label\":\"-\",\"type\":\"foundation.electrical.electrical\"},{\"id\":\"H\",\"label\":\"H\",\"type\":\"foundation.thermal.thermal\"}],\"Top\":[]}"
  Busbar (DC){,1..5} (6 alike) : ee_lib/Connectors & References/Busbar (DC)  n_nodes=ee.enum.connectors.busbar_number_of_connections.one  VRated=1e3 V  measurement_type=ee.enum.measurementType.instantaneous  averaging_period=1e-2 s  show_ps=ee.enum.connectors.busbar_measurement.false
      settings: InternalSimscapePortConfiguration="{\"Bottom\":[],\"Left\":[{\"id\":\"p1\",\"label\":\"1+\",\"type\":\"foundation.electrical.electrical\"},{\"id\":\"n1\",\"label\":\"1-\",\"type\":\"foundation.electrical.electrical\"}],\"Right\":[],\"Top\":[]}"
  Pos : PMIOPort  Side=Left
  Thermal : PMIOPort  Port=2  Side=Right
  Neg : PMIOPort  Port=3  Side=Right
  connections:
  Battery (System-Level)3/RConn1 -- Busbar (DC)3/LConn1
  Battery (System-Level)1/RConn1 -- Busbar (DC)1/LConn1
  Battery (System-Level)5/RConn2 -- Battery (System-Level)4/RConn2 -- Battery (System-Level)3/RConn2 -- Battery (System-Level)2/RConn2 -- Battery (System-Level)1/RConn2 -- Battery (System-Level)/RConn2 -- Thermal/RConn1
  Battery (System-Level)3/LConn1 -- Busbar (DC)2/LConn2
  Battery (System-Level)5/RConn1 -- Busbar (DC)5/LConn1
  Battery (System-Level)/RConn1 -- Busbar (DC)/LConn1
  Battery (System-Level)4/LConn1 -- Busbar (DC)3/LConn2
  Battery (System-Level)2/RConn1 -- Busbar (DC)2/LConn1
  Busbar (DC)5/LConn2 -- Neg/RConn1
  Battery (System-Level)/LConn1 -- Pos/RConn1
  Battery (System-Level)2/LConn1 -- Busbar (DC)1/LConn2
  Battery (System-Level)4/RConn1 -- Busbar (DC)4/LConn1
  Battery (System-Level)5/LConn1 -- Busbar (DC)4/LConn2
  Battery (System-Level)1/LConn1 -- Busbar (DC)/LConn2

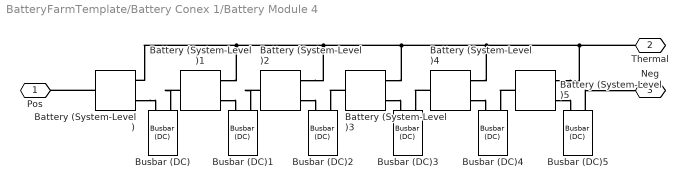
== system BatteryFarmTemplate/Battery Conex 1/Battery Module 4 ==
  Battery (System-Level){,1..5} (6 alike) : sdl_lib/Sources/Battery (System-Level)  Vnom=3.1 V  R1=0.021 Ohm  prm_AH=sdl.enum.InfiniteFinite.Infinite  AH=50 A*hr  V1=11.5 V  AH1=25 A*hr  prm_R2=sdl.enum.DisabledEnabled.Disabled  R2=2000 Ohm  thermal_port=simscape.enum.thermaleffects.model  thermal_mass=30000 J/K  i_specify=off  i_priority=None  i=0 A  i_nominal_specify=off  i_nominal_unit=A  i_nominal_value=1  v_specify=off  v_priority=None  v=0 V  v_nominal_specify=off  v_nominal_unit=V  v_nominal_value=1  charge_specify=off  charge_priority=High  charge=50 A*hr  charge_nominal_specify=off  charge_nominal_unit=A*hr  charge_nominal_value=1  temperature_specify=off  temperature_priority=High  temperature=300 K  temperature_nominal_specify=off  temperature_nominal_unit=K  temperature_nominal_value=1
      settings: InternalSimscapePortConfiguration="{\"Bottom\":[],\"Left\":[{\"id\":\"p\",\"label\":\"+\",\"type\":\"foundation.electrical.electrical\"}],\"Right\":[{\"id\":\"n\",\"label\":\"-\",\"type\":\"foundation.electrical.electrical\"},{\"id\":\"H\",\"label\":\"H\",\"type\":\"foundation.thermal.thermal\"}],\"Top\":[]}"
  Busbar (DC){,1..5} (6 alike) : ee_lib/Connectors & References/Busbar (DC)  n_nodes=ee.enum.connectors.busbar_number_of_connections.one  VRated=1e3 V  measurement_type=ee.enum.measurementType.instantaneous  averaging_period=1e-2 s  show_ps=ee.enum.connectors.busbar_measurement.false
      settings: InternalSimscapePortConfiguration="{\"Bottom\":[],\"Left\":[{\"id\":\"p1\",\"label\":\"1+\",\"type\":\"foundation.electrical.electrical\"},{\"id\":\"n1\",\"label\":\"1-\",\"type\":\"foundation.electrical.electrical\"}],\"Right\":[],\"Top\":[]}"
  Pos : PMIOPort  Side=Left
  Thermal : PMIOPort  Port=2  Side=Right
  Neg : PMIOPort  Port=3  Side=Right
  connections:
  Battery (System-Level)3/RConn1 -- Busbar (DC)3/LConn1
  Battery (System-Level)1/RConn1 -- Busbar (DC)1/LConn1
  Battery (System-Level)5/RConn2 -- Battery (System-Level)4/RConn2 -- Battery (System-Level)3/RConn2 -- Battery (System-Level)2/RConn2 -- Battery (System-Level)1/RConn2 -- Battery (System-Level)/RConn2 -- Thermal/RConn1
  Battery (System-Level)3/LConn1 -- Busbar (DC)2/LConn2
  Battery (System-Level)5/RConn1 -- Busbar (DC)5/LConn1
  Battery (System-Level)/RConn1 -- Busbar (DC)/LConn1
  Battery (System-Level)4/LConn1 -- Busbar (DC)3/LConn2
  Battery (System-Level)2/RConn1 -- Busbar (DC)2/LConn1
  Busbar (DC)5/LConn2 -- Neg/RConn1
  Battery (System-Level)/LConn1 -- Pos/RConn1
  Battery (System-Level)2/LConn1 -- Busbar (DC)1/LConn2
  Battery (System-Level)4/RConn1 -- Busbar (DC)4/LConn1
  Battery (System-Level)5/LConn1 -- Busbar (DC)4/LConn2
  Battery (System-Level)1/LConn1 -- Busbar (DC)/LConn2

== system BatteryFarmTemplate/Battery Conex 1/Battery Module 5 ==
  Battery (System-Level){,1..5} (6 alike) : sdl_lib/Sources/Battery (System-Level)  Vnom=3.1 V  R1=0.021 Ohm  prm_AH=sdl.enum.InfiniteFinite.Infinite  AH=50 A*hr  V1=11.5 V  AH1=25 A*hr  prm_R2=sdl.enum.DisabledEnabled.Disabled  R2=2000 Ohm  thermal_port=simscape.enum.thermaleffects.model  thermal_mass=30000 J/K  i_specify=off  i_priority=None  i=0 A  i_nominal_specify=off  i_nominal_unit=A  i_nominal_value=1  v_specify=off  v_priority=None  v=0 V  v_nominal_specify=off  v_nominal_unit=V  v_nominal_value=1  charge_specify=off  charge_priority=High  charge=50 A*hr  charge_nominal_specify=off  charge_nominal_unit=A*hr  charge_nominal_value=1  temperature_specify=off  temperature_priority=High  temperature=300 K  temperature_nominal_specify=off  temperature_nominal_unit=K  temperature_nominal_value=1
      settings: InternalSimscapePortConfiguration="{\"Bottom\":[],\"Left\":[{\"id\":\"p\",\"label\":\"+\",\"type\":\"foundation.electrical.electrical\"}],\"Right\":[{\"id\":\"n\",\"label\":\"-\",\"type\":\"foundation.electrical.electrical\"},{\"id\":\"H\",\"label\":\"H\",\"type\":\"foundation.thermal.thermal\"}],\"Top\":[]}"
  Busbar (DC){,1..5} (6 alike) : ee_lib/Connectors & References/Busbar (DC)  n_nodes=ee.enum.connectors.busbar_number_of_connections.one  VRated=1e3 V  measurement_type=ee.enum.measurementType.instantaneous  averaging_period=1e-2 s  show_ps=ee.enum.connectors.busbar_measurement.false
      settings: InternalSimscapePortConfiguration="{\"Bottom\":[],\"Left\":[{\"id\":\"p1\",\"label\":\"1+\",\"type\":\"foundation.electrical.electrical\"},{\"id\":\"n1\",\"label\":\"1-\",\"type\":\"foundation.electrical.electrical\"}],\"Right\":[],\"Top\":[]}"
  Pos : PMIOPort  Side=Left
  Thermal : PMIOPort  Port=2  Side=Right
  Neg : PMIOPort  Port=3  Side=Right
  connections:
  Battery (System-Level)3/RConn1 -- Busbar (DC)3/LConn1
  Battery (System-Level)1/RConn1 -- Busbar (DC)1/LConn1
  Battery (System-Level)5/RConn2 -- Battery (System-Level)4/RConn2 -- Battery (System-Level)3/RConn2 -- Battery (System-Level)2/RConn2 -- Battery (System-Level)1/RConn2 -- Battery (System-Level)/RConn2 -- Thermal/RConn1
  Battery (System-Level)3/LConn1 -- Busbar (DC)2/LConn2
  Battery (System-Level)5/RConn1 -- Busbar (DC)5/LConn1
  Battery (System-Level)/RConn1 -- Busbar (DC)/LConn1
  Battery (System-Level)4/LConn1 -- Busbar (DC)3/LConn2
  Battery (System-Level)2/RConn1 -- Busbar (DC)2/LConn1
  Busbar (DC)5/LConn2 -- Neg/RConn1
  Battery (System-Level)/LConn1 -- Pos/RConn1
  Battery (System-Level)2/LConn1 -- Busbar (DC)1/LConn2
  Battery (System-Level)4/RConn1 -- Busbar (DC)4/LConn1
  Battery (System-Level)5/LConn1 -- Busbar (DC)4/LConn2
  Battery (System-Level)1/LConn1 -- Busbar (DC)/LConn2

== system BatteryFarmTemplate/Battery Conex 1/Battery Module 6 ==
  Battery (System-Level){,1..5} (6 alike) : sdl_lib/Sources/Battery (System-Level)  Vnom=3.1 V  R1=0.021 Ohm  prm_AH=sdl.enum.InfiniteFinite.Infinite  AH=50 A*hr  V1=11.5 V  AH1=25 A*hr  prm_R2=sdl.enum.DisabledEnabled.Disabled  R2=2000 Ohm  thermal_port=simscape.enum.thermaleffects.model  thermal_mass=30000 J/K  i_specify=off  i_priority=None  i=0 A  i_nominal_specify=off  i_nominal_unit=A  i_nominal_value=1  v_specify=off  v_priority=None  v=0 V  v_nominal_specify=off  v_nominal_unit=V  v_nominal_value=1  charge_specify=off  charge_priority=High  charge=50 A*hr  charge_nominal_specify=off  charge_nominal_unit=A*hr  charge_nominal_value=1  temperature_specify=off  temperature_priority=High  temperature=300 K  temperature_nominal_specify=off  temperature_nominal_unit=K  temperature_nominal_value=1
      settings: InternalSimscapePortConfiguration="{\"Bottom\":[],\"Left\":[{\"id\":\"p\",\"label\":\"+\",\"type\":\"foundation.electrical.electrical\"}],\"Right\":[{\"id\":\"n\",\"label\":\"-\",\"type\":\"foundation.electrical.electrical\"},{\"id\":\"H\",\"label\":\"H\",\"type\":\"foundation.thermal.thermal\"}],\"Top\":[]}"
  Busbar (DC){,1..5} (6 alike) : ee_lib/Connectors & References/Busbar (DC)  n_nodes=ee.enum.connectors.busbar_number_of_connections.one  VRated=1e3 V  measurement_type=ee.enum.measurementType.instantaneous  averaging_period=1e-2 s  show_ps=ee.enum.connectors.busbar_measurement.false
      settings: InternalSimscapePortConfiguration="{\"Bottom\":[],\"Left\":[{\"id\":\"p1\",\"label\":\"1+\",\"type\":\"foundation.electrical.electrical\"},{\"id\":\"n1\",\"label\":\"1-\",\"type\":\"foundation.electrical.electrical\"}],\"Right\":[],\"Top\":[]}"
  Pos : PMIOPort  Side=Left
  Thermal : PMIOPort  Port=2  Side=Right
  Neg : PMIOPort  Port=3  Side=Right
  connections:
  Battery (System-Level)3/RConn1 -- Busbar (DC)3/LConn1
  Battery (System-Level)1/RConn1 -- Busbar (DC)1/LConn1
  Battery (System-Level)5/RConn2 -- Battery (System-Level)4/RConn2 -- Battery (System-Level)3/RConn2 -- Battery (System-Level)2/RConn2 -- Battery (System-Level)1/RConn2 -- Battery (System-Level)/RConn2 -- Thermal/RConn1
  Battery (System-Level)3/LConn1 -- Busbar (DC)2/LConn2
  Battery (System-Level)5/RConn1 -- Busbar (DC)5/LConn1
  Battery (System-Level)/RConn1 -- Busbar (DC)/LConn1
  Battery (System-Level)4/LConn1 -- Busbar (DC)3/LConn2
  Battery (System-Level)2/RConn1 -- Busbar (DC)2/LConn1
  Busbar (DC)5/LConn2 -- Neg/RConn1
  Battery (System-Level)/LConn1 -- Pos/RConn1
  Battery (System-Level)2/LConn1 -- Busbar (DC)1/LConn2
  Battery (System-Level)4/RConn1 -- Busbar (DC)4/LConn1
  Battery (System-Level)5/LConn1 -- Busbar (DC)4/LConn2
  Battery (System-Level)1/LConn1 -- Busbar (DC)/LConn2

== system BatteryFarmTemplate/Battery Conex 1/Battery Module 7 ==
  Battery (System-Level){,1..5} (6 alike) : sdl_lib/Sources/Battery (System-Level)  Vnom=3.1 V  R1=0.021 Ohm  prm_AH=sdl.enum.InfiniteFinite.Infinite  AH=50 A*hr  V1=11.5 V  AH1=25 A*hr  prm_R2=sdl.enum.DisabledEnabled.Disabled  R2=2000 Ohm  thermal_port=simscape.enum.thermaleffects.model  thermal_mass=30000 J/K  i_specify=off  i_priority=None  i=0 A  i_nominal_specify=off  i_nominal_unit=A  i_nominal_value=1  v_specify=off  v_priority=None  v=0 V  v_nominal_specify=off  v_nominal_unit=V  v_nominal_value=1  charge_specify=off  charge_priority=High  charge=50 A*hr  charge_nominal_specify=off  charge_nominal_unit=A*hr  charge_nominal_value=1  temperature_specify=off  temperature_priority=High  temperature=300 K  temperature_nominal_specify=off  temperature_nominal_unit=K  temperature_nominal_value=1
      settings: InternalSimscapePortConfiguration="{\"Bottom\":[],\"Left\":[{\"id\":\"p\",\"label\":\"+\",\"type\":\"foundation.electrical.electrical\"}],\"Right\":[{\"id\":\"n\",\"label\":\"-\",\"type\":\"foundation.electrical.electrical\"},{\"id\":\"H\",\"label\":\"H\",\"type\":\"foundation.thermal.thermal\"}],\"Top\":[]}"
  Busbar (DC){,1..5} (6 alike) : ee_lib/Connectors & References/Busbar (DC)  n_nodes=ee.enum.connectors.busbar_number_of_connections.one  VRated=1e3 V  measurement_type=ee.enum.measurementType.instantaneous  averaging_period=1e-2 s  show_ps=ee.enum.connectors.busbar_measurement.false
      settings: InternalSimscapePortConfiguration="{\"Bottom\":[],\"Left\":[{\"id\":\"p1\",\"label\":\"1+\",\"type\":\"foundation.electrical.electrical\"},{\"id\":\"n1\",\"label\":\"1-\",\"type\":\"foundation.electrical.electrical\"}],\"Right\":[],\"Top\":[]}"
  Pos : PMIOPort  Side=Left
  Thermal : PMIOPort  Port=2  Side=Right
  Neg : PMIOPort  Port=3  Side=Right
  connections:
  Battery (System-Level)3/RConn1 -- Busbar (DC)3/LConn1
  Battery (System-Level)1/RConn1 -- Busbar (DC)1/LConn1
  Battery (System-Level)5/RConn2 -- Battery (System-Level)4/RConn2 -- Battery (System-Level)3/RConn2 -- Battery (System-Level)2/RConn2 -- Battery (System-Level)/RConn2 -- Battery (System-Level)1/RConn2 -- Thermal/RConn1
  Battery (System-Level)3/LConn1 -- Busbar (DC)2/LConn2
  Battery (System-Level)5/RConn1 -- Busbar (DC)5/LConn1
  Battery (System-Level)/RConn1 -- Busbar (DC)/LConn1
  Battery (System-Level)4/LConn1 -- Busbar (DC)3/LConn2
  Battery (System-Level)2/RConn1 -- Busbar (DC)2/LConn1
  Busbar (DC)5/LConn2 -- Neg/RConn1
  Battery (System-Level)/LConn1 -- Pos/RConn1
  Battery (System-Level)2/LConn1 -- Busbar (DC)1/LConn2
  Battery (System-Level)4/RConn1 -- Busbar (DC)4/LConn1
  Battery (System-Level)5/LConn1 -- Busbar (DC)4/LConn2
  Battery (System-Level)1/LConn1 -- Busbar (DC)/LConn2
